simulink model "lab1a"  (R2018a)
settings: Solver=FixedStepDiscrete  StartTime=0.0  StopTime=10.0  FixedStep=dt  RelTol=1e-3  EnableMultiTasking=on
values from neighbouring files (symbols this model uses):
  A = (1-f)/T    (= 20)    [lab1a_plot.m]
  f = 0.9    [lab1a_plot.m]
  Kd = 0.5    [lab1a_plot.m]
  Kd_2 = 0.5    [lab1a_plot.m]
  Kp = 100    [lab1a_plot.m]
  Kp_2 = 200    [lab1a_plot.m]
libraries: legoev3lib x4
settings Model: SimulationMode=external  ExtModeTrigDuration=2  Creator=jacobdelrosario  LastModifiedBy=richardboone
settings SolverCC: PositivePriorityOrder=on
settings OptimizationCC: EnhancedBackFolding=on  PassReuseOutputArgsAs=Individual arguments  MaxStackSize=64  OptimizeBlockOrder=speed  DifferentSizesBufferReuse=on  OptimizationCustomize=off
settings DebuggingCC: ParameterTunabilityLossMsg=error
settings HardwareCC: ProdBitPerPointer=32  ProdBitPerSizeT=32  ProdBitPerPtrDiffT=32  ProdLargestAtomicInteger=Long  ProdWordSize=32  ProdHWDeviceType=ARM Compatible->ARM 9
settings SFSimCC: MATLABDynamicMemAlloc=off
settings RTWCC: SystemTargetFile=ert.tlc  HardwareBoard=LEGO MINDSTORMS EV3  TLCOptions="-aInlineSetEventsForThisBaseRateFcn=TLC_FALSE -aSuppressMultiTaskScheduler=TLC_FALSE  -aRateBasedStepFcn=0"  TemplateMakefile=ert_default_tmf  GenerateReport=on  Toolchain=Sourcery G++ Lite v2009q3  IncludeHyperlinkInReport=on  LaunchReport=on  GenerateTraceInfo=on  GenerateTraceReport=on  GenerateTraceReportSl=on  GenerateTraceReportSf=on  GenerateTraceReportEml=on
settings CodeAppCC: ForceParamTrailComments=on  IgnoreCustomStorageClasses=off  OperatorAnnotations=on  SimulinkDataObjDesc=on  SFDataObjDesc=on  InsertBlockDesc=on
settings ERTTargetCC: SupportContinuousTime=on  SupportVariableSizeSignals=on

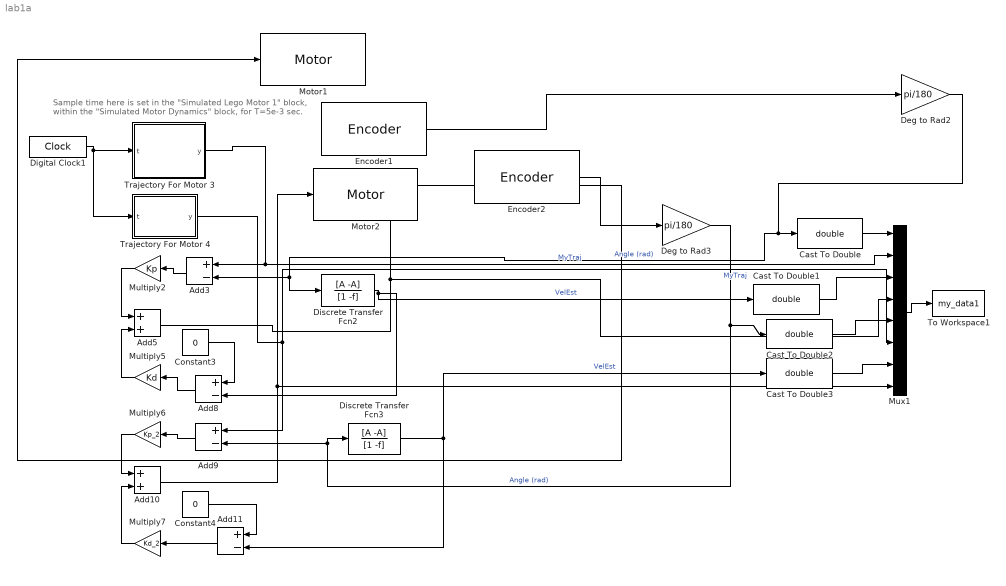
== system lab1a ==
  note: Sample time here is set in the "Simulated Lego Motor 1" block,
      | within the "Simulated Motor Dynamics" block, for T=5e-3 sec.
  Add10 : Sum
  Add{3,8..9,11} (4 alike) : Sum  Inputs=+-
  Add5 : Sum
  Cast To Double{,1..3} (4 alike) : DataTypeConversion  OutDataTypeStr=double
  Constant3 : Constant  Value=0
  Constant4 : Constant  Value=0
  Deg to Rad2 : Gain  Gain=pi/180
  Deg to Rad3 : Gain  Gain=pi/180
  Digital Clock1 : DigitalClock  SampleTime=5e-3
  Discrete Transfer Fcn2 : DiscreteTransferFcn  Numerator=[A -A]  Denominator=[1 -f]  SampleTime=0.005
  Discrete Transfer Fcn3 : DiscreteTransferFcn  Numerator=[A -A]  Denominator=[1 -f]  SampleTime=0.005
  Encoder1 : legoev3lib/Encoder  portNumber=A  opMode=No reset  sampleTime=dt
      settings: SourceProductName=Simulink Support Package for LEGO MINDSTORMS EV3 Hardware  SourceProductBaseCode=LEGOEV3
  Encoder2 : legoev3lib/Encoder  portNumber=D  opMode=No reset  sampleTime=dt
      settings: SourceProductName=Simulink Support Package for LEGO MINDSTORMS EV3 Hardware  SourceProductBaseCode=LEGOEV3
  Motor1 : legoev3lib/Motor  sportNumber=A  sstopAction=Brake
  Motor2 : legoev3lib/Motor  sportNumber=D  sstopAction=Brake
  Multiply2 : Gain  Gain=Kp
  Multiply5 : Gain  Gain=Kd
  Multiply6 : Gain  Gain=Kp_2
  Multiply7 : Gain  Gain=Kd_2
  Mux1 : Mux  Inputs=8
  To Workspace1 : ToWorkspace  VariableName=my_data1  SaveFormat=Structure With Time  SampleTime=-1
  Trajectory For Motor 3 : MATLAB Function  TreatAsAtomicUnit=on
  Trajectory For Motor 4 : MATLAB Function  TreatAsAtomicUnit=on
  wires:
  Encoder1/1 -> Deg to Rad2/1
  Add5/1 -> Motor1/1, Mux1/4
  Trajectory For Motor 3/1(y) -> Mux1/2, Add3/1  "MyTraj"
  Deg to Rad2/1 -> Add3/2, Discrete Transfer Fcn2/1, Cast To Double/1  "Angle (rad)"
  Multiply7/1 -> Add10/2
  Digital Clock1/1 -> Trajectory For Motor 3/1(t), Trajectory For Motor 4/1(t)
  Constant3/1 -> Add8/1
  Add9/1 -> Multiply6/1
  Trajectory For Motor 4/1(y) -> Mux1/6, Add9/1  "MyTraj"
  Add3/1 -> Multiply2/1
  Discrete Transfer Fcn3/1 -> Cast To Double3/1, Add11/2  "VelEst"
  Mux1/1 -> To Workspace1/1
  Constant4/1 -> Add11/1
  Multiply6/1 -> Add10/1
  Discrete Transfer Fcn2/1 -> Add8/2, Cast To Double1/1  "VelEst"
  Multiply2/1 -> Add5/1
  Add11/1 -> Multiply7/1
  Deg to Rad3/1 -> Add9/2, Discrete Transfer Fcn3/1, Cast To Double2/1  "Angle (rad)"
  Multiply5/1 -> Add5/2
  Add8/1 -> Multiply5/1
  Cast To Double/1 -> Mux1/1
  Cast To Double1/1 -> Mux1/3
  Add10/1 -> Mux1/8, Motor2/1
  Encoder2/1 -> Deg to Rad3/1
  Cast To Double2/1 -> Mux1/5
  Cast To Double3/1 -> Mux1/7

== matlab function lab1a/Trajectory For Motor 3 ==
  data: t input; y output

function y = MyTrajectory(t)
%L1 = 11.2;
%L2 = 8;
L1 = 14.5;
L2 = 10.5;
%% Define y(t) as a desired TRAJECTORY as a function of TIME
if 1
    h = 10 + 2.5*sqrt(3);
    ti = [0 10 12 22 24 34 36 46 200];
    ti = ti/5;
    xi = [7.5 7.5 12.5 12.5 10 10 7.5 7.5 7.5];
    yi = [10 10 10 10 h h 10 10 10];
    set = 0;
    y = 0;
    for i=1:8
        if ti(i) <= t && ti(i+1) > t
            set = 1;
            partdist = (t - ti(i))/(ti(i+1) - ti(i));
            %xloc = (partdist * (xi(i+1) - xi(i))) + xi(i);
            %yloc = (partdist * (yi(i+1) - yi(i))) + yi(i);
            xloc = xi(i);
            yloc = yi(i);
            y = TranslateToThetaTwo(xloc, yloc, L1, L2);
        end
    end
    if set == 0
        y = 0;
    end
elseif 0
    %% Example 1: a step, which starts at t=1 second
    t_start = 1; % have the step occur at t = t_start
    StepMag = 0.4; % For a step in RAW INPUT to motor (open loop)
    % StepMag = 0.3; % for a step in RADIANS, as a TRAJECTORY (closed loop)
    % Here, this the VALUE TO THE MOTOR (analogous to open-loop voltage)
    if t>=t_start
        y = StepMag;
    else
        y = 0;
    end
    
    
elseif 0
    %% Example 2: a trajectory, in RADIANS, for the motor to follow
    t_start = 1;
    A = 0.3; % In RADIANS
    w = 2*2*pi;
    if t>=t_start
        t_use = t - t_start;
        y = A * sin(w*t_use);
    else
        y = 0;
    end
    
elseif 0
    %% Example 3: using interp1() and some waypoints
    ti = [0 1 2 3 100];
    yi = [0 0 20 -30 -30]*(pi/180);
    y = interp1(ti,yi,t);  % LINEAR INTERPOLATION, as a REFERENCE
else
    %% Example 4: using half-cosine function, for smooth transitions
    ypts = [0 0 30 -20 0 0]*pi/180;
    tpts = [0 1 2 3 4 10];
    if t < tpts(2)
        y1 = ypts(1); y2 = ypts(2);
        t1 = tpts(1); t2 = tpts(2);
    elseif t < tpts(3)
        y1 = ypts(2); y2 = ypts(3);
        t1 = tpts(2); t2 = tpts(3);
    elseif t < tpts(4)
        y1 = ypts(3); y2 = ypts(4);
        t1 = tpts(3); t2 = tpts(4);
    elseif t < tpts(5)
        y1 = ypts(4); y2 = ypts(5); % Hold at SAME VALUE
        t1 = tpts(4); t2 = tpts(5);
    else
        y1 = ypts(5); y2 = ypts(6);
        t1 = tpts(5); t2 = tpts(6);
    end
    tPhase = (t-t1) / (t2-t1);  % goes from 0 to 1
    cosVal = cos(pi * tPhase);  % cos(pi*tPhase) will go from 1 to -1...
    y = y1 + (y2 - y1) * (.5 * (1-cosVal)); % cosine shape, going
    % from 0 to 1, as tPhase goes from 0 to pi.
end
end



function theta_two = TranslateToThetaTwo(x, y, L1, L2)
    top = (L1^2) +  (L2^2) - ((x^2) + (y^2));
    bottom = 2 * L1 * L2;
    theta_two =  pi - acos(top/bottom);
end

function theta_one = TranslateToThetaOne(x, y, L1, L2)
    theta_two = TranslateToThetaTwo(x, y, L1, L2);
    left = atan(y/x);
    right = atan((L2 * sin(theta_two))/(L1 + (L2 * cos(theta_two))));
    theta_one = left - right;
end

== matlab function lab1a/Trajectory For Motor 4 ==
  data: t input; y output

function y = MyTrajectory(t)
%L1 = 11.2;
%L2 = 8;
L1 = 14.5;
L2 = 10.5;
%% Define y(t) as a desired TRAJECTORY as a function of TIME
if 1
    h = 10 + 2.5*sqrt(3);
    ti = [0 10 12 22 24 34 36 46 200];
    ti = ti/5;
    xi = [7.5 7.5 12.5 12.5 10 10 7.5 7.5 7.5];
    yi = [10 10 10 10 h h 10 10 10];
    set = 0;
    y = 0;
    for i=1:8
        if ti(i) <= t && ti(i+1) > t
            set = 1;
            partdist = (t - ti(i))/(ti(i+1) - ti(i));
            %xloc = (partdist * (xi(i+1) - xi(i))) + xi(i);
            %yloc = (partdist * (yi(i+1) - yi(i))) + yi(i);
            xloc = xi(i);
            yloc = yi(i);
            y = TranslateToThetaOne(xloc, yloc, L1, L2);
        end
    end
    if set == 0
        y = 0;
    end    
elseif 0
    %% Example 1: a step, which starts at t=1 second
    t_start = 1; % have the step occur at t = t_start
    StepMag = 100; % For a step in RAW INPUT to motor (open loop)
    % StepMag = 0.3; % for a step in RADIANS, as a TRAJECTORY (closed loop)
    % Here, this the VALUE TO THE MOTOR (analogous to open-loop voltage)
    if t>=t_start
        y = StepMag;
    else
        y = 0;
    end
    
    
elseif 0
    %% Example 2: a trajectory, in RADIANS, for the motor to follow
    t_start = 1;
    A = 0.3; % In RADIANS
    w = 2*2*pi;
    if t>=t_start
        t_use = t - t_start;
        y = A * sin(w*t_use);
    else
        y = 0;
    end
    
elseif 0
    %% Example 3: using interp1() and some waypoints
    ti = [0 1 2 3 100];
    yi = [0 0 20 -30 -30]*(pi/180);
    y = interp1(ti,yi,t);  % LINEAR INTERPOLATION, as a REFERENCE
else
    %% Example 4: using half-cosine function, for smooth transitions
    ypts = [0 0 30 -20 0 0]*pi/180;
    tpts = [0 1 2 3 4 10];
    if t < tpts(2)
        y1 = ypts(1); y2 = ypts(2);
        t1 = tpts(1); t2 = tpts(2);
    elseif t < tpts(3)
        y1 = ypts(2); y2 = ypts(3);
        t1 = tpts(2); t2 = tpts(3);
    elseif t < tpts(4)
        y1 = ypts(3); y2 = ypts(4);
        t1 = tpts(3); t2 = tpts(4);
    elseif t < tpts(5)
        y1 = ypts(4); y2 = ypts(5); % Hold at SAME VALUE
        t1 = tpts(4); t2 = tpts(5);
    else
        y1 = ypts(5); y2 = ypts(6);
        t1 = tpts(5); t2 = tpts(6);
    end
    tPhase = (t-t1) / (t2-t1);  % goes from 0 to 1
    cosVal = cos(pi * tPhase);  % cos(pi*tPhase) will go from 1 to -1...
    y = y1 + (y2 - y1) * (.5 * (1-cosVal)); % cosine shape, going
    % from 0 to 1, as tPhase goes from 0 to pi.
end
end



function theta_two = TranslateToThetaTwo(x, y, L1, L2)
    top = (L1^2) +  (L2^2) - ((x^2) + (y^2));
    bottom = 2 * L1 * L2;
    theta_two =  pi - acos(top/bottom);
end

function theta_one = TranslateToThetaOne(x, y, L1, L2)
    theta_two = TranslateToThetaTwo(x, y, L1, L2);
    left = atan(y/x);
    right = atan((L2 * sin(theta_two))/(L1 + (L2 * cos(theta_two))));
    theta_one = left - right;
end
